simulink model "ex02_model"  (R2023a)
settings: Solver=FixedStepDiscrete  StartTime=0.0  StopTime=length(x)*Ts  RelTol=1e-3
undefined symbols (not defined in the file): h, M, Ts
libraries: dspsrcs4 x1
settings Model: Creator=daniele  LastModifiedBy=daniele
settings SolverCC: AlgebraicLoopSolver=TrustRegion
settings DataIOCC: ReturnWorkspaceOutputs=off
settings DebuggingCC: UnconnectedInputMsg=warning  UnconnectedOutputMsg=warning  UnconnectedLineMsg=warning  ArithmeticOperatorsInVariantConditions=warning
settings ModelReferenceCC: EnableRefExpFcnMdlSchedulingChecks=on
settings SFSimCC: CustomCodeUndefinedFunction=UseInterfaceOnly

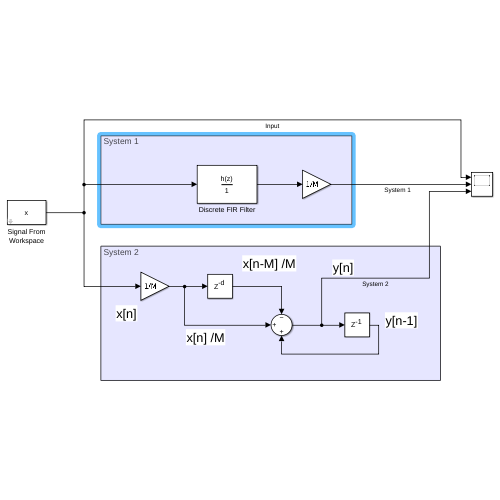
[thumbnail: Simulink's stored preview of the top-level diagram]
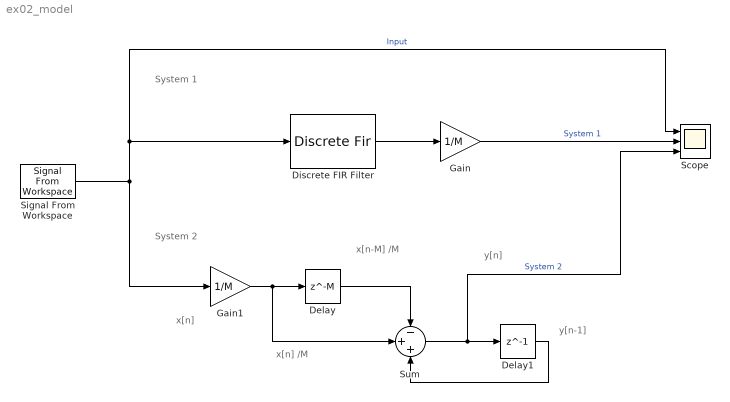
== system ex02_model ==
  note: System 2
  note: System 1
  note: y[n]
  note: x[n]
  note: x[n] /M
  note: x[n-M] /M
  note: y[n-1]
  Delay : Delay  DelayLength=M
  Delay1 : Delay  DelayLength=1
  Discrete FIR Filter : DiscreteFir  Coefficients=h
  Gain : Gain  Gain=1/M
  Gain1 : Gain  Gain=1/M
  Scope : Scope  NumInputPorts=3
  Signal From Workspace : dspsrcs4/Signal From Workspace  X=x  Ts=Ts  nsamps=1  OutputAfterFinalValue=Setting to zero  ignoreOrWarnInputAndFrameLengths=off  OutputFrames=off
  Sum : Sum  Inputs=-++
  wires:
  Discrete FIR Filter/1 -> Gain/1
  Gain/1 -> Scope/2  "System 1"
  Gain1/1 -> Sum/2, Delay/1
  Signal From Workspace/1 -> Gain1/1, Discrete FIR Filter/1, Scope/1  "Input"
  Delay/1 -> Sum/1
  Delay1/1 -> Sum/3
  Sum/1 -> Scope/3, Delay1/1  "System 2"
